simulink model "EKF_aoa_acc"  (R2019a)
settings: Solver=FixedStepAuto  StartTime=0.0  StopTime=300  FixedStep=0.2  RelTol=1e-3
libraries: simulink_extras x1
settings Model: Creator=phand  LastModifiedBy=phand

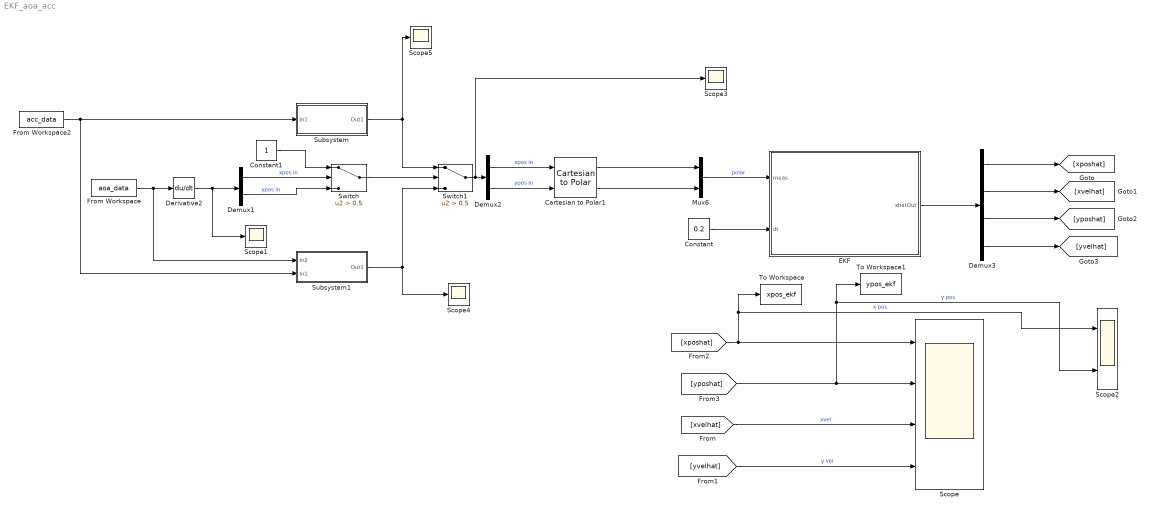
== system EKF_aoa_acc ==
  Cartesian to Polar1 : simulink_extras/Transformations/Cartesian to Polar
      settings: SourceProductName=Simulink
  Constant : Constant  Value=0.2
  Constant1 : Constant
  Demux1 : Demux  Outputs=2
  Demux2 : Demux  Outputs=2
  Demux3 : Demux
  Derivative2 : Derivative
  "EKF " : MATLAB Function  TreatAsAtomicUnit=on
  From Workspace : FromWorkspace  VariableName=aoa_data  SampleTime=0
  From Workspace2 : FromWorkspace  VariableName=acc_data  SampleTime=0
  Mux6 : Mux  Inputs=2
  Scope : Scope  NumInputPorts=4
  Scope{1,3..5} (4 alike) : Scope
  Scope2 : Scope  NumInputPorts=2
  Subsystem : Subsystem
  Subsystem1 : Subsystem
  Switch : Switch  Criteria=u2 > Threshold  Threshold=0.5
  Switch1 : Switch  Criteria=u2 > Threshold  Threshold=0.5
  To Workspace : ToWorkspace  VariableName=xpos_ekf  SampleTime=-1
  To Workspace1 : ToWorkspace  VariableName=ypos_ekf  SampleTime=-1
  wires:
  Constant/1 -> "EKF "/2(dt)
  Demux3/4 -> [yvelhat]
  Demux3/2 -> [xvelhat]
  "EKF "/1(xhatOut) -> Demux3/1
  Demux3/3 -> [yposhat]
  Demux3/1 -> [xposhat]
  From Workspace/1 -> Subsystem1/1(In2), Derivative2/1
  [xposhat] -> Scope2/1, To Workspace/1, Scope/1  "x pos"
  [yposhat] -> Scope2/2, To Workspace1/1, Scope/2  "y pos"
  [xvelhat] -> Scope/3  "xvel"
  [yvelhat] -> Scope/4  "y vel"
  Demux2/1 -> Cartesian to Polar1/1  "xpos in"
  Demux2/2 -> Cartesian to Polar1/2  "ypos in"
  Cartesian to Polar1/1 -> Mux6/1
  Cartesian to Polar1/2 -> Mux6/2
  Derivative2/1 -> Scope1/1, Demux1/1
  From Workspace2/1 -> Subsystem1/2(In1), Subsystem/1(In1)
  Switch/1 -> Switch1/2
  Constant1/1 -> Switch/1
  Demux1/1 -> Switch/2  "xpos in"
  Demux1/2 -> Switch/3  "ypos in"
  Subsystem/1(Out1) -> Scope5/1, Switch1/1
  Subsystem1/1(Out1) -> Scope4/1, Switch1/3
  Switch1/1 -> Scope3/1, Demux2/1
  Mux6/1 -> "EKF "/1(meas)  "polar"

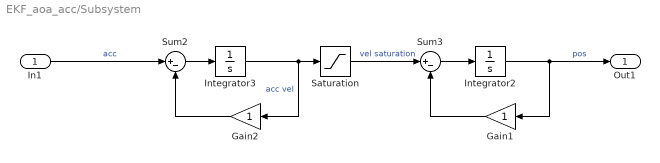
== system EKF_aoa_acc/Subsystem ==
  In1 : Inport
  Gain1 : Gain
  Gain2 : Gain
  Integrator2 : Integrator
  Integrator3 : Integrator
  Saturation : Saturate  UpperLimit=7  LowerLimit=-7
  Sum2 : Sum  Inputs=|+-
  Sum3 : Sum  Inputs=|+-
  Out1 : Outport
  wires:
  In1/1 -> Sum2/1  "acc"
  Gain2/1 -> Sum2/2
  Sum3/1 -> Integrator2/1
  Integrator3/1 -> Gain2/1, Saturation/1  "acc vel"
  Integrator2/1 -> Out1/1, Gain1/1  "pos"
  Gain1/1 -> Sum3/2
  Sum2/1 -> Integrator3/1
  Saturation/1 -> Sum3/1  "vel saturation"

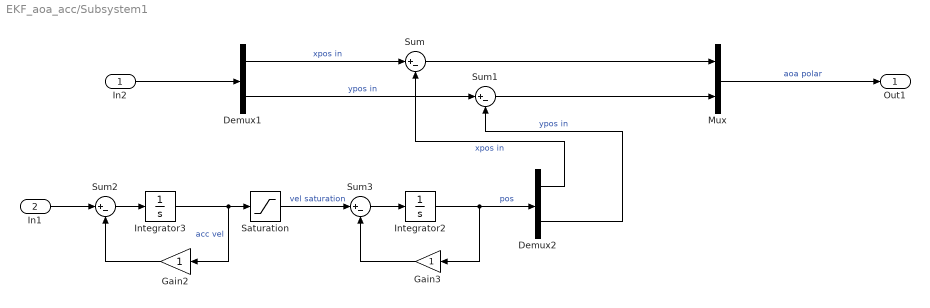
== system EKF_aoa_acc/Subsystem1 ==
  In2 : Inport
  In1 : Inport  Port=2
  Demux1 : Demux  Outputs=2
  Demux2 : Demux  Outputs=2
  Gain2 : Gain
  Gain3 : Gain
  Integrator2 : Integrator
  Integrator3 : Integrator
  Mux : Mux  Inputs=2
  Saturation : Saturate  UpperLimit=7  LowerLimit=-7
  Sum{,1..3} (4 alike) : Sum  Inputs=|+-
  Out1 : Outport
  wires:
  Mux/1 -> Out1/1  "aoa polar"
  Sum1/1 -> Mux/2
  Demux2/2 -> Sum1/2  "ypos in"
  Demux2/1 -> Sum/2  "xpos in"
  Demux1/2 -> Sum1/1  "ypos in"
  Sum/1 -> Mux/1
  Sum2/1 -> Integrator3/1
  Gain3/1 -> Sum3/2
  Saturation/1 -> Sum3/1  "vel saturation"
  Integrator3/1 -> Gain2/1, Saturation/1  "acc vel"
  Sum3/1 -> Integrator2/1
  Integrator2/1 -> Demux2/1, Gain3/1  "pos"
  Gain2/1 -> Sum2/2
  In1/1 -> Sum2/1
  Demux1/1 -> Sum/1  "xpos in"
  In2/1 -> Demux1/1

== matlab function EKF_aoa_acc/EKF  ==
  settings: updateMethod=DISCRETE
  data: meas input; xhatOut output; dt input
function xhatOut = EKF(meas, dt)
% This Embedded MATLAB Function implements an extended Kalman filter used
% for object tracking.
%
% The states of the process are given by
% x = [x_position; x_velocity; y_position; y_velocity];
%
% and the measurements are given by
% y = [range; bearing]
%
% where 
% range = sqrt(x_position^2 + y_position^2)
% bearing = atan2(y_position/x_position)

% Author: Phil Goddard (phil@goddardconsulting.ca)
% Date: Q2, 2011.

% Define storage for the variables that need to persist
% between time periods.
persistent P xhat Q R
if isempty(P)
    %[xvel, yvel] = acc_init(35);
    %[xpos, ypos] = aoa_init(35);
    %[xinit, yinit] = acc_init(35);
    %[xposinit, yposinit] = aoa_init(35);
    xpos = 3;
    %xvel = 3.5;
    ypos = 4.2;
    %yvel = 1.2;
    
    % First time through the code so do some initialization
    xhat = [-1.255; 0.1; 1.11; 0.1];
    %xhat = [-900;80;950;20];
    P = zeros(4,4);
    Q =  diag([0.3 0.6 0.3 0.6]);
    R =  diag([0.25 0.25]);
end
% Calculate the Jacobians for the state and measurement equations
F = [1 dt 0 0;0 1 0 0;0 0 1 dt;0 0 0 1];
rangeHat = sqrt(xhat(1)^2+xhat(3)^2);
bearingHat = atan2(xhat(3),xhat(1));
yhat = [rangeHat; bearingHat]; 
H = [cos(bearingHat) 0 sin(bearingHat) 0;
    -sin(bearingHat)/rangeHat 0 cos(bearingHat)/rangeHat 0];

% Propogate the state and covariance matrices
xhat = F*xhat;
P = F*P*F' + Q;

% Calculate the Kalman gain
K = P*H'/(H*P*H' + R);

% Calculate the measurement residual
resid = meas - yhat;

% Update the state and covariance estimates
xhat = xhat + K*resid;
P = (eye(size(K,1))-K*H)*P;

% Post the results
xhatOut = xhat;
